simulink model "code_sim_ele"  (R2022a)
settings: Solver=FixedStepAuto  StartTime=0.0  StopTime=40  FixedStep=0.1  RelTol=1e-3
libraries: simulink x5
settings Model: Creator=AlaiC  LastModifiedBy=AlaiC
settings RTWCC: GenCodeOnly=on  PackageGeneratedCodeAndArtifacts=on  PackageName=simulated_elevator.zip
settings GRTTargetCC: MatFileLogging=off

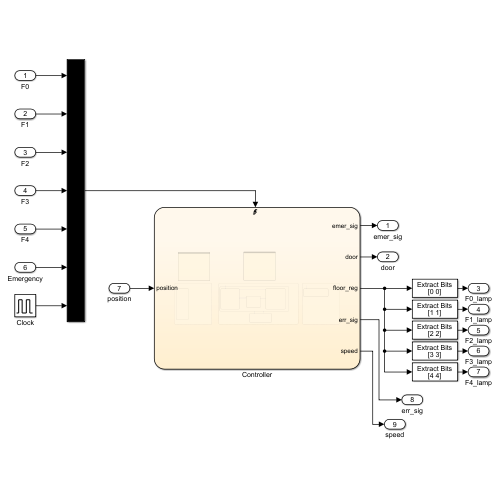
[thumbnail: Simulink's stored preview of the top-level diagram]
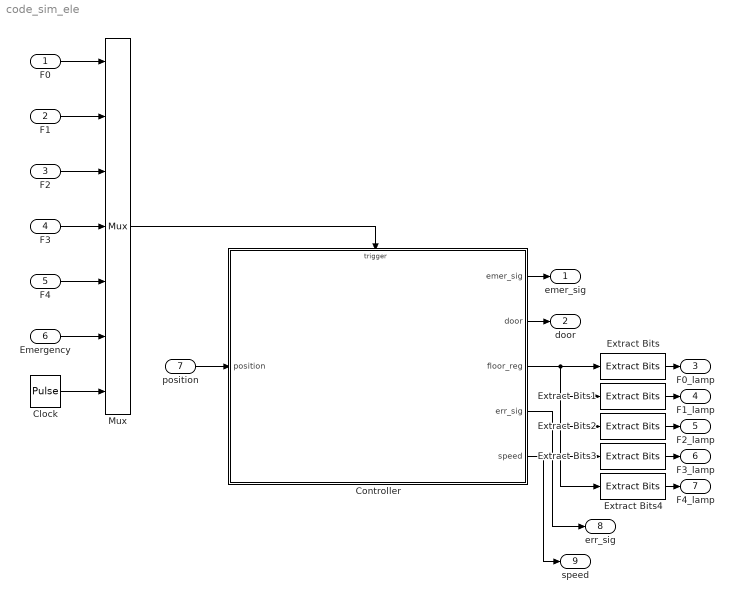
== system code_sim_ele ==
  F0 : Inport
  F1 : Inport  Port=2
  F2 : Inport  Port=3
  F3 : Inport  Port=4
  F4 : Inport  Port=5
  Emergency : Inport  Port=6
  position : Inport  Port=7
  Clock : DiscretePulseGenerator  PulseType=Time based  Period=0.2  PulseWidth=50
  Controller : Stateflow chart  TreatAsAtomicUnit=on
  Extract Bits : simulink/Logic and Bit Operations/Extract Bits  bitsToExtract=Range of bits  numBits=8  bitIdxRange=[0 0]  outScalingMode=Preserve fixed-point scaling
  Extract Bits1 : simulink/Logic and Bit Operations/Extract Bits  bitsToExtract=Range of bits  numBits=8  bitIdxRange=[1 1]  outScalingMode=Preserve fixed-point scaling
  Extract Bits2 : simulink/Logic and Bit Operations/Extract Bits  bitsToExtract=Range of bits  numBits=8  bitIdxRange=[2 2]  outScalingMode=Preserve fixed-point scaling
  Extract Bits3 : simulink/Logic and Bit Operations/Extract Bits  bitsToExtract=Range of bits  numBits=8  bitIdxRange=[3 3]  outScalingMode=Preserve fixed-point scaling
  Extract Bits4 : simulink/Logic and Bit Operations/Extract Bits  bitsToExtract=Range of bits  numBits=8  bitIdxRange=[4 4]  outScalingMode=Preserve fixed-point scaling
  Mux : Mux  Inputs=7
  emer_sig : Outport
  door : Outport  Port=2
  F0_lamp : Outport  Port=3
  F1_lamp : Outport  Port=4
  F2_lamp : Outport  Port=5
  F3_lamp : Outport  Port=6
  F4_lamp : Outport  Port=7
  err_sig : Outport  Port=8
  speed : Outport  Port=9
  wires:
  Mux/1 -> Controller/Trigger
  F0/1 -> Mux/1
  F1/1 -> Mux/2
  F2/1 -> Mux/3
  F3/1 -> Mux/4
  F4/1 -> Mux/5
  Emergency/1 -> Mux/6
  Extract Bits/1 -> F0_lamp/1
  Extract Bits1/1 -> F1_lamp/1
  Extract Bits2/1 -> F2_lamp/1
  Controller/3(floor_reg) -> Extract Bits3/1, Extract Bits4/1, Extract Bits2/1, Extract Bits1/1, Extract Bits/1
  Extract Bits3/1 -> F3_lamp/1
  Extract Bits4/1 -> F4_lamp/1
  Controller/1(emer_sig) -> emer_sig/1
  Controller/2(door) -> door/1
  Controller/5(speed) -> speed/1
  Clock/1 -> Mux/7
  Controller/4(err_sig) -> err_sig/1
  position/1 -> Controller/1(position)

== stateflow chart code_sim_ele/Controller ==
  state speed_o = setspeed(dir, init_pos, pos, des) [function]
    (default) -> (junction 519)
    (junction 519) -> (junction 528) [order 1] : [dir > 0]
    (junction 519) -> (junction 526) [order 2] : [dir < 0]
    (junction 528) -> (junction 530) [order 1] : [pos - init_pos < 0.2 ]
        | {speed_o = 0.3*(pos - init_pos + 0.01)*5}
    (junction 526) -> (junction 538) [order 1] : [init_pos - pos < 0.2]
        | {speed_o = -0.3*(init_pos - pos + 0.01)*5}
    (junction 528) -> (junction 532) [order 2]
    (junction 519) -> (junction 558) [order 3] : {speed_o = 0;}
    (junction 526) -> (junction 540) [order 2]
    (junction 532) -> (junction 534) [order 1] : [des - pos >= 0.2]
        | {speed_o = 0.3}
    (junction 540) -> (junction 542) [order 1] : [pos - des >= 0.2]
        | {speed_o = -0.3}
    (junction 532) -> (junction 536) [order 2] : {speed_o = 0.3*(des - pos)*5}
    (junction 540) -> (junction 544) [order 2] : {speed_o = -0.3*(pos - des)*5}
  state des = ElevatorDes (dir, floor_r, pos) [function]
    (default) -> (junction 487)
    (junction 487) -> (junction 489) [order 2]
    (junction 489) -> (junction 491) [order 1] : [pos == 0 || pos == 1 || pos == 2 || pos == 3 || pos == 4]
        | {des = -1;}
    (junction 489) -> (junction 493) [order 2]
    (junction 487) -> (junction 204) [order 1] : [floor_r ~= 0]
    (junction 493) -> (junction 495) [order 1] : [dir >=0]{des = ceil(pos);}
    (junction 493) -> (junction 497) [order 2] : {des = floor(pos);}
    (junction 205) -> (junction 398) [order 1] : [pos >= 3 && bitget(floor_r,5)]
        | {des = 4;}
    (junction 204) -> (junction 205) [order 1] : [dir >= 0]
    (junction 442) -> (junction 474) [order 1] : [pos <= 1 && bitget(floor_r,1)]
        | {des = 0;}
    (junction 204) -> (junction 442) [order 2]
    (junction 205) -> (junction 399) [order 2]
    (junction 442) -> (junction 448) [order 2]
    (junction 399) -> (junction 401) [order 1] : [pos >= 2 && bitget(floor_r,4)]
        | {des = 3;}
    (junction 448) -> (junction 478) [order 1] : [pos <= 2 && bitget(floor_r,2)]
        | {des = 1;}
    (junction 399) -> (junction 403) [order 2]
    (junction 448) -> (junction 476) [order 2]
    (junction 403) -> (junction 405) [order 1] : [pos >= 2 && bitget(floor_r,5)]
        | {des = 4;}
    (junction 476) -> (junction 451) [order 1] : [pos <= 2 && bitget(floor_r,1)]
        | {des = 0;}
    (junction 403) -> (junction 407) [order 2]
    (junction 476) -> (junction 483) [order 2]
    (junction 407) -> (junction 409) [order 1] : [pos >= 1 && bitget(floor_r,3)]
        | {des = 2;}
    (junction 483) -> (junction 485) [order 1] : [pos <= 3 && bitget(floor_r,3)]
        | {des = 2;}
    (junction 407) -> (junction 411) [order 2]
    (junction 483) -> (junction 445) [order 2]
    (junction 411) -> (junction 413) [order 1] : [pos >= 1 && bitget(floor_r,4)]
        | {des = 3;}
    (junction 445) -> (junction 447) [order 1] : [pos <= 3 && bitget(floor_r,2)]
        | {des = 1;}
    (junction 411) -> (junction 415) [order 2]
    (junction 445) -> (junction 455) [order 2]
    (junction 415) -> (junction 417) [order 1] : [pos >= 1 && bitget(floor_r,5)]
        | {des = 4;}
    (junction 455) -> (junction 456) [order 1] : [pos <= 3 && bitget(floor_r,1)]
        | {des = 0;}
    (junction 415) -> (junction 428) [order 2]
    (junction 455) -> (junction 466) [order 2]
    (junction 428) -> (junction 424) [order 1] : [pos >= 0 && bitget(floor_r,2)]
        | {des = 1;}
    (junction 466) -> (junction 461) [order 1] : [pos <= 4 && bitget(floor_r,4)]
        | {des = 3;}
    (junction 428) -> (junction 431) [order 2]
    (junction 466) -> (junction 462) [order 2]
    (junction 431) -> (junction 433) [order 1] : [pos >= 0 && bitget(floor_r,3)]
        | {des = 2;}
    (junction 462) -> (junction 465) [order 1] : [pos <= 4 && bitget(floor_r,3)]
        | {des = 2;}
    (junction 431) -> (junction 420) [order 2]
    (junction 462) -> (junction 457) [order 2]
    (junction 420) -> (junction 422) [order 1] : [pos >= 0 && bitget(floor_r,4)]
        | {des = 3;}
    (junction 457) -> (junction 470) [order 1] : [pos <= 4 && bitget(floor_r,2)]
        | {des = 1;}
    (junction 420) -> (junction 426) [order 2]
    (junction 457) -> (junction 463) [order 2]
    (junction 426) -> (junction 427) [order 1] : [pos >= 0 && bitget(floor_r,5)]
        | {des = 4;}
    (junction 463) -> (junction 460) [order 1] : [pos <= 4 && bitget(floor_r,1)]
        | {des = 0;}
    (junction 426) -> (junction 436) [order 2]
    (junction 463) -> (junction 452) [order 2]
    (junction 436) -> (junction 438) [order 1] : [bitget(floor_reg,1)]
        | {des = 0;}
    (junction 452) -> (junction 481) [order 1] : [bitget(floor_reg,5)]
        | {des = 4;}
    (junction 436) -> (junction 440) [order 2] : {des = -1;}
    (junction 452) -> (junction 472) [order 2] : {des = -1;}
  state ErrDetection [parallel]
    settings: executionOrder=3
    state default
      en:
      err_sig = false;
      du:
      if position < -0.1 || position > 4.1 || abs(position - pre_position) >= 0.3
      err_sig = true;
      else
      pre_position = position;
      end
    (default) -> default : {pre_position = 0;}
  state InputHandler [parallel]
    settings: executionOrder=1
    state button
      on emergency:
      emer_sig = ~emer_sig;
      on F0:
      if ~bitget(floor_reg,1)
      floor_reg = bitset(floor_reg,1,1);
      F0_preTime = -1;
      else
      if getSimulationTime() - F0_preTime <= 1
      floor_reg = bitset(floor_reg,1,0);
      end
      F0_preTime = getSimulationTime();
      end
      on F1:
      if ~bitget(floor_reg,2)
      floor_reg = bitset(floor_reg,2,1);
      F1_preTime = -1;
      else
      if getSimulationTime() - F1_preTime <= 1
      floor_reg = bitset(floor_reg,2,0);
      end
      F1_preTime = getSimulationTime();
      end
      on F2:
      if ~bitget(floor_reg,3)
      floor_reg = bitset(floor_reg,3,1);
      F2_preTime = -1;
      else
      if getSimulationTime() - F2_preTime <= 1
      floor_reg = bitset(floor_reg,3,0);
      end
      F2_preTime = getSimulationTime();
      end
      on F3:
      if ~bitget(floor_reg,4)
      floor_reg = bitset(floor_reg,4,1);
      F3_preTime = -1;
      else
      if getSimulationTime() - F3_preTime <= 1
      floor_reg = bitset(floor_reg,4,0);
      end
      F3_preTime = getSimulationTime();
      end
      on F4:
      if ~bitget(floor_reg,5)
      floor_reg = bitset(floor_reg,5,1);
      F4_preTime = -1;
      else
      if getSimulationTime() - F4_preTime <= 1
      floor_reg = bitset(floor_reg,5,0);
      end
      F4_preTime = getSimulationTime();
      end
    (default) -> button : {floor_reg = 0b00000;
        | emer_sig = false;
        | F0_preTime = -1;
        | F1_preTime = -1;
        | F2_preTime = -1;
        | F3_preTime = -1;
        | F4_preTime = -1;}
  state LogicController [parallel]
    settings: executionOrder=2
    state DEFAULT
      state Idel
        en:
        pre_dir = cur_dir;
        cur_dir = 0;
        door = false;
        speed = 0;
        on TIC:
        if floor_reg ~= 0
        destination = ElevatorDes(pre_dir,floor_reg,position);
        else
        destination = -1;
        cur_dir = 0;
        end
        if destination ~= -1 && position > destination - 0.1 && position < destination +0.1
        if destination == 0
        floor_reg = bitset(floor_reg,1,0);
        elseif destination == 1
        floor_reg = bitset(floor_reg,2,0);
        elseif destination == 2
        floor_reg = bitset(floor_reg,3,0);
        elseif destination == 3
        floor_reg = bitset(floor_reg,4,0);
        elseif destination == 4
        floor_reg = bitset(floor_reg,5,0);
        end
        cur_dir = 0;
        door_open = 1;
        elseif destination ~= -1 && destination > position + 0.1
        cur_dir = 1;
        elseif destination ~= -1 && destination < position - 0.1
        cur_dir = -1;
        else
        cur_dir = 0;
        end
      state Run
        en:
        init_position = position;
        on TIC:
        if position > destination - 0.1 && position < destination +0.1
        if destination == 0
        floor_reg = bitset(floor_reg,1,0);
        elseif destination == 1
        floor_reg = bitset(floor_reg,2,0);
        elseif destination == 2
        floor_reg = bitset(floor_reg,3,0);
        elseif destination == 3
        floor_reg = bitset(floor_reg,4,0);
        elseif destination == 4
        floor_reg = bitset(floor_reg,5,0);
        end
        door_open = 1;
        speed = 0;
        elseif abs(position - destination) < 0.2
        destination = destination;
        speed = setspeed(cur_dir, init_position, position, destination);
        else
        destination = ElevatorDes(cur_dir,floor_reg,position);
        speed = setspeed(cur_dir, init_position, position, destination);
        end
      state Open
        en:
        door_open = 0;
        door = true;
        speed = 0;
        on TIC:
        if position > -0.1 && position < 0.1 && bitget(floor_reg,1)
        floor_reg = bitset(floor_reg,1,0);
        elseif position > 0.9 && position < 1.1 && bitget(floor_reg,2)
        floor_reg = bitset(floor_reg,2,0);
        elseif position > 1.9 && position < 2.1 && bitget(floor_reg,3)
        floor_reg = bitset(floor_reg,3,0);
        elseif position > 2.9 && position < 3.1 && bitget(floor_reg,4)
        floor_reg = bitset(floor_reg,4,0);
        elseif position > 3.9 && position < 4.1 && bitget(floor_reg,5)
        floor_reg = bitset(floor_reg,5,0);
        end
        ex:
        door = false;
      (default) -> Idel : {cur_dir = 0;
          | door_open = 0;}
      Idel -> Run [order 2] : [cur_dir == 1 || cur_dir == -1]
      Idel -> Open [order 1] : [door_open]
      Run -> Open : [door_open]
      Open -> Idel : after(5,sec)
    state EMER_ERR
      en:
      speed = 0;
    (default) -> DEFAULT
    DEFAULT -> EMER_ERR : [emer_sig || err_sig]
    EMER_ERR -> DEFAULT : [~emer_sig && ~err_sig]
  data: dir function_input; init_pos function_input; pos function_input; des function_input; speed_o function_output; dir function_input; floor_r function_input; pos function_input; des function_output; emer_sig output boolean; F0_preTime local; F1_preTime local; F2_preTime local; F3_preTime local; F4_preTime local; position input double; cur_dir local; door output boolean; floor_reg output; err_sig output boolean; destination local; pre_dir local; door_open local; speed output double; init_position local double; pre_position local; E_destination local
  events: F0 input RISING_EDGE_EVENT; F1 input RISING_EDGE_EVENT; F2 input RISING_EDGE_EVENT; F3 input RISING_EDGE_EVENT; F4 input RISING_EDGE_EVENT; emergency input RISING_EDGE_EVENT; TIC input RISING_EDGE_EVENT
